simulink model "case8"  (R2024b)
settings: Solver=FixedStepAuto  StartTime=0  StopTime=1  FixedStep=1e-7  RelTol=1e-3
values from neighbouring files (symbols this model uses):
  SG_D_1_D = 0.01056    [IEEE9_case_parameters.m]    (also in case1_parameters.m; case2_parameters.m; case3_parameters.m; case4_parameters.m)
  SG_D_1_EnableSaturation = 0    [IEEE9_case_parameters.m]    (also in case1_parameters.m; case2_parameters.m; case3_parameters.m; case4_parameters.m)
  SG_D_1_f0 = 60    [IEEE9_case_parameters.m]    (also in case1_parameters.m; case2_parameters.m; case3_parameters.m; case4_parameters.m)
  SG_D_1_H = 7.5    [IEEE9_case_parameters.m]    (also in case1_parameters.m; case2_parameters.m; case3_parameters.m; case4_parameters.m)
  SG_D_1_K_A = 20    [IEEE9_case_parameters.m]    (also in case1_parameters.m; case2_parameters.m; case3_parameters.m; case4_parameters.m)
  SG_D_1_K_E = 1.000000e+1    (= 10)    [IEEE9_case_parameters.m]    (also in case1_parameters.m; case2_parameters.m; case3_parameters.m; case4_parameters.m)
  SG_D_1_K_F = 2.363    [IEEE9_case_parameters.m]    (also in case1_parameters.m; case2_parameters.m; case3_parameters.m; case4_parameters.m)
  SG_D_1_K_s = 0.5    [IEEE9_case_parameters.m]    (also in case1_parameters.m = 5; case2_parameters.m = 5; case3_parameters.m = 5; case4_parameters.m = 5)
  SG_D_1_R_a = 0.001088    [IEEE9_case_parameters.m]    (also in case1_parameters.m; case2_parameters.m; case3_parameters.m; case4_parameters.m)
  SG_D_1_S_A = 1    [IEEE9_case_parameters.m]    (also in case1_parameters.m; case2_parameters.m; case3_parameters.m; case4_parameters.m)
  SG_D_1_S_B = 0.103    [IEEE9_case_parameters.m]    (also in case1_parameters.m; case2_parameters.m; case3_parameters.m; case4_parameters.m)
  SG_D_1_S_N = 10.659857    [IEEE9_case_parameters.m]    (also in case1_parameters.m; case2_parameters.m; case3_parameters.m; case4_parameters.m)
  SG_D_1_SpeedPara = 200    [IEEE9_case_parameters.m]    (also in case1_parameters.m; case2_parameters.m; case3_parameters.m; case4_parameters.m)
  SG_D_1_T_0 = 0.720173    [IEEE9_case_parameters.m]    (also in case1_parameters.m = 0.755522; case2_parameters.m = 0.808931; case3_parameters.m = 0.869402; case4_parameters.m = 0.729316)
  SG_D_1_T_1 = 0.3    [IEEE9_case_parameters.m]    (also in case1_parameters.m; case2_parameters.m; case3_parameters.m; case4_parameters.m)
  SG_D_1_T_2 = 0.05    [IEEE9_case_parameters.m]    (also in case1_parameters.m; case2_parameters.m; case3_parameters.m; case4_parameters.m)
  SG_D_1_T_3 = 0.02    [IEEE9_case_parameters.m]    (also in case1_parameters.m; case2_parameters.m; case3_parameters.m; case4_parameters.m)
  SG_D_1_T_4 = 0.005    [IEEE9_case_parameters.m]    (also in case1_parameters.m; case2_parameters.m; case3_parameters.m; case4_parameters.m)
  SG_D_1_T_A = 0.02    [IEEE9_case_parameters.m]    (also in case1_parameters.m; case2_parameters.m; case3_parameters.m; case4_parameters.m)
  SG_D_1_T_dd = 8.000000e+0    (= 8)    [IEEE9_case_parameters.m]    (also in case1_parameters.m; case2_parameters.m; case3_parameters.m; case4_parameters.m)
  SG_D_1_T_ddd = 0.04    [IEEE9_case_parameters.m]    (also in case1_parameters.m; case2_parameters.m; case3_parameters.m; case4_parameters.m)
  SG_D_1_T_E = 0.314    [IEEE9_case_parameters.m]    (also in case1_parameters.m; case2_parameters.m; case3_parameters.m; case4_parameters.m)
  SG_D_1_T_F = 0.35    [IEEE9_case_parameters.m]    (also in case1_parameters.m; case2_parameters.m; case3_parameters.m; case4_parameters.m)
  SG_D_1_T_qd = 0.8    [IEEE9_case_parameters.m]    (also in case1_parameters.m; case2_parameters.m; case3_parameters.m; case4_parameters.m)
  SG_D_1_T_qdd = 0.02    [IEEE9_case_parameters.m]    (also in case1_parameters.m; case2_parameters.m; case3_parameters.m; case4_parameters.m)
  SG_D_1_T_speed = 0.1    [IEEE9_case_parameters.m]    (also in case1_parameters.m = 200; case2_parameters.m = 200; case3_parameters.m = 200; case4_parameters.m = 200)
  SG_D_1_T_w = 0.5    [IEEE9_case_parameters.m]    (also in case1_parameters.m; case2_parameters.m; case3_parameters.m; case4_parameters.m)
  SG_D_1_V_ref = 1.990276    [IEEE9_case_parameters.m]    (also in case1_parameters.m = 2.042296; case2_parameters.m = 2.051388; case3_parameters.m = 2.089584; case4_parameters.m = 2.01845)
  SG_D_1_w_ref = 376.991118    [IEEE9_case_parameters.m]    (also in case1_parameters.m; case2_parameters.m; case3_parameters.m; case4_parameters.m)
  SG_D_1_wb = 6.000000e+1    (= 60)    [IEEE9_case_parameters.m]    (also in case1_parameters.m; case2_parameters.m; case3_parameters.m; case4_parameters.m)
  SG_D_1_x_d = 1.9    [IEEE9_case_parameters.m]    (also in case1_parameters.m; case2_parameters.m; case3_parameters.m; case4_parameters.m)
  SG_D_1_x_dd = 0.302    [IEEE9_case_parameters.m]    (also in case1_parameters.m; case2_parameters.m; case3_parameters.m; case4_parameters.m)
  SG_D_1_x_ddd = 0.204    [IEEE9_case_parameters.m]    (also in case1_parameters.m; case2_parameters.m; case3_parameters.m; case4_parameters.m)
  SG_D_1_x_l = 0.05    [IEEE9_case_parameters.m]    (also in case1_parameters.m; case2_parameters.m; case3_parameters.m; case4_parameters.m)
  SG_D_1_x_q = 1.3    [IEEE9_case_parameters.m]    (also in case1_parameters.m; case2_parameters.m; case3_parameters.m; case4_parameters.m)
  SG_D_1_x_qd = 0.5    [IEEE9_case_parameters.m]    (also in case1_parameters.m; case2_parameters.m; case3_parameters.m; case4_parameters.m)
  SG_D_1_x_qdd = 0.3    [IEEE9_case_parameters.m]    (also in case1_parameters.m; case2_parameters.m; case3_parameters.m; case4_parameters.m)
  SG_D_2_D = 0.02    [IEEE9_case_parameters.m]    (also in case1_parameters.m; case2_parameters.m; case3_parameters.m; case4_parameters.m)
  SG_D_2_EnableSaturation = 0    [IEEE9_case_parameters.m]    (also in case1_parameters.m; case2_parameters.m; case3_parameters.m; case4_parameters.m)
  SG_D_2_f0 = 60    [IEEE9_case_parameters.m]    (also in case1_parameters.m; case2_parameters.m; case3_parameters.m; case4_parameters.m)
  SG_D_2_H = 8.000000e+0    (= 8)    [IEEE9_case_parameters.m]    (also in case1_parameters.m; case2_parameters.m; case3_parameters.m; case4_parameters.m)
  SG_D_2_K_A = 20    [IEEE9_case_parameters.m]    (also in case1_parameters.m; case2_parameters.m; case3_parameters.m; case4_parameters.m)
  SG_D_2_K_E = 1.000000e+1    (= 10)    [IEEE9_case_parameters.m]    (also in case1_parameters.m; case2_parameters.m; case3_parameters.m; case4_parameters.m)
  SG_D_2_K_F = 2.363    [IEEE9_case_parameters.m]    (also in case1_parameters.m; case2_parameters.m; case3_parameters.m; case4_parameters.m)
  SG_D_2_K_s = 0.5    [IEEE9_case_parameters.m]    (also in case1_parameters.m = 4; case2_parameters.m = 4; case3_parameters.m = 4; case4_parameters.m = 4)
  SG_D_2_R_a = 0.001088    [IEEE9_case_parameters.m]    (also in case1_parameters.m; case2_parameters.m; case3_parameters.m; case4_parameters.m)
  SG_D_2_S_A = 1    [IEEE9_case_parameters.m]    (also in case1_parameters.m; case2_parameters.m; case3_parameters.m; case4_parameters.m)
  SG_D_2_S_B = 0.103    [IEEE9_case_parameters.m]    (also in case1_parameters.m; case2_parameters.m; case3_parameters.m; case4_parameters.m)
  SG_D_2_S_N = 10.659857    [IEEE9_case_parameters.m]    (also in case1_parameters.m; case2_parameters.m; case3_parameters.m; case4_parameters.m)
  SG_D_2_SpeedPara = 200    [IEEE9_case_parameters.m]    (also in case1_parameters.m; case2_parameters.m; case3_parameters.m; case4_parameters.m)
  SG_D_2_T_0 = 1.632913    [IEEE9_case_parameters.m]    (also in case1_parameters.m = 1.632925; case2_parameters.m = 1.632915; case3_parameters.m = 1.632914; case4_parameters.m = 1.632927)
  SG_D_2_T_1 = 0.2    [IEEE9_case_parameters.m]    (also in case1_parameters.m; case2_parameters.m; case3_parameters.m; case4_parameters.m)
  SG_D_2_T_2 = 0.05    [IEEE9_case_parameters.m]    (also in case1_parameters.m; case2_parameters.m; case3_parameters.m; case4_parameters.m)
  SG_D_2_T_3 = 0.02    [IEEE9_case_parameters.m]    (also in case1_parameters.m; case2_parameters.m; case3_parameters.m; case4_parameters.m)
  SG_D_2_T_4 = 0.005    [IEEE9_case_parameters.m]    (also in case1_parameters.m; case2_parameters.m; case3_parameters.m; case4_parameters.m)
  SG_D_2_T_A = 0.02    [IEEE9_case_parameters.m]    (also in case1_parameters.m; case2_parameters.m; case3_parameters.m; case4_parameters.m)
  SG_D_2_T_dd = 7.9    [IEEE9_case_parameters.m]    (also in case1_parameters.m; case2_parameters.m; case3_parameters.m; case4_parameters.m)
  SG_D_2_T_ddd = 0.04    [IEEE9_case_parameters.m]    (also in case1_parameters.m; case2_parameters.m; case3_parameters.m; case4_parameters.m)
  SG_D_2_T_E = 0.314    [IEEE9_case_parameters.m]    (also in case1_parameters.m; case2_parameters.m; case3_parameters.m; case4_parameters.m)
  SG_D_2_T_F = 0.35    [IEEE9_case_parameters.m]    (also in case1_parameters.m; case2_parameters.m; case3_parameters.m; case4_parameters.m)
  SG_D_2_T_qd = 0.8    [IEEE9_case_parameters.m]    (also in case1_parameters.m; case2_parameters.m; case3_parameters.m; case4_parameters.m)
  SG_D_2_T_qdd = 0.015    [IEEE9_case_parameters.m]    (also in case1_parameters.m; case2_parameters.m; case3_parameters.m; case4_parameters.m)
  SG_D_2_T_speed = 0.1    [IEEE9_case_parameters.m]    (also in case1_parameters.m = 150; case2_parameters.m = 150; case3_parameters.m = 150; case4_parameters.m = 150)
  SG_D_2_T_w = 0.35    [IEEE9_case_parameters.m]    (also in case1_parameters.m; case2_parameters.m; case3_parameters.m; case4_parameters.m)
  SG_D_2_V_ref = 2.58547    [IEEE9_case_parameters.m]    (also in case1_parameters.m = 2.597896; case2_parameters.m = 2.587136; case3_parameters.m = 2.586042; case4_parameters.m = 2.599679)
  SG_D_2_w_ref = 376.991118    [IEEE9_case_parameters.m]    (also in case1_parameters.m; case2_parameters.m; case3_parameters.m; case4_parameters.m)
  SG_D_2_wb = 6.000000e+1    (= 60)    [IEEE9_case_parameters.m]    (also in case1_parameters.m; case2_parameters.m; case3_parameters.m; case4_parameters.m)
  SG_D_2_x_d = 1.8    [IEEE9_case_parameters.m]    (also in case1_parameters.m; case2_parameters.m; case3_parameters.m; case4_parameters.m)
  SG_D_2_x_dd = 0.302    [IEEE9_case_parameters.m]    (also in case1_parameters.m; case2_parameters.m; case3_parameters.m; case4_parameters.m)
  SG_D_2_x_ddd = 0.204    [IEEE9_case_parameters.m]    (also in case1_parameters.m; case2_parameters.m; case3_parameters.m; case4_parameters.m)
  SG_D_2_x_l = 0.05    [IEEE9_case_parameters.m]    (also in case1_parameters.m; case2_parameters.m; case3_parameters.m; case4_parameters.m)
  SG_D_2_x_q = 1.25    [IEEE9_case_parameters.m]    (also in case1_parameters.m; case2_parameters.m; case3_parameters.m; case4_parameters.m)
  SG_D_2_x_qd = 0.5    [IEEE9_case_parameters.m]    (also in case1_parameters.m; case2_parameters.m; case3_parameters.m; case4_parameters.m)
  SG_D_2_x_qdd = 0.3    [IEEE9_case_parameters.m]    (also in case1_parameters.m; case2_parameters.m; case3_parameters.m; case4_parameters.m)
  SG_D_3_D = 0.02    [IEEE9_case_parameters.m]    (also in case1_parameters.m; case2_parameters.m; case3_parameters.m; case4_parameters.m)
  SG_D_3_EnableSaturation = 0    [IEEE9_case_parameters.m]    (also in case1_parameters.m; case2_parameters.m; case3_parameters.m; case4_parameters.m)
  SG_D_3_f0 = 60    [IEEE9_case_parameters.m]    (also in case1_parameters.m; case2_parameters.m; case3_parameters.m; case4_parameters.m)
  SG_D_3_H = 7.7    [IEEE9_case_parameters.m]    (also in case1_parameters.m; case2_parameters.m; case3_parameters.m; case4_parameters.m)
  SG_D_3_K_A = 20    [IEEE9_case_parameters.m]    (also in case1_parameters.m; case2_parameters.m; case3_parameters.m; case4_parameters.m)
  SG_D_3_K_E = 1.000000e+1    (= 10)    [IEEE9_case_parameters.m]    (also in case1_parameters.m; case2_parameters.m; case3_parameters.m; case4_parameters.m)
  SG_D_3_K_F = 2.363    [IEEE9_case_parameters.m]    (also in case1_parameters.m; case2_parameters.m; case3_parameters.m; case4_parameters.m)
  SG_D_3_K_s = 0.2    [IEEE9_case_parameters.m]    (also in case1_parameters.m = 2; case2_parameters.m = 2; case3_parameters.m = 2; case4_parameters.m = 2)
  SG_D_3_R_a = 0.001088    [IEEE9_case_parameters.m]    (also in case1_parameters.m; case2_parameters.m; case3_parameters.m; case4_parameters.m)
  SG_D_3_S_A = 1    [IEEE9_case_parameters.m]    (also in case1_parameters.m; case2_parameters.m; case3_parameters.m; case4_parameters.m)
  SG_D_3_S_B = 0.103    [IEEE9_case_parameters.m]    (also in case1_parameters.m; case2_parameters.m; case3_parameters.m; case4_parameters.m)
  SG_D_3_S_N = 10.659857    [IEEE9_case_parameters.m]    (also in case1_parameters.m; case2_parameters.m; case3_parameters.m; case4_parameters.m)
  SG_D_3_SpeedPara = 200    [IEEE9_case_parameters.m]    (also in case1_parameters.m; case2_parameters.m; case3_parameters.m; case4_parameters.m)
  SG_D_3_T_0 = 0.850788    [IEEE9_case_parameters.m]    (also in case1_parameters.m = 0.850786; case2_parameters.m = 0.850787; case3_parameters.m; case4_parameters.m = 0.850786)
  SG_D_3_T_1 = 0.2    [IEEE9_case_parameters.m]    (also in case1_parameters.m; case2_parameters.m; case3_parameters.m; case4_parameters.m)
  SG_D_3_T_2 = 0.05    [IEEE9_case_parameters.m]    (also in case1_parameters.m; case2_parameters.m; case3_parameters.m; case4_parameters.m)
  SG_D_3_T_3 = 0.02    [IEEE9_case_parameters.m]    (also in case1_parameters.m; case2_parameters.m; case3_parameters.m; case4_parameters.m)
  SG_D_3_T_4 = 0.005    [IEEE9_case_parameters.m]    (also in case1_parameters.m; case2_parameters.m; case3_parameters.m; case4_parameters.m)
  SG_D_3_T_A = 0.02    [IEEE9_case_parameters.m]    (also in case1_parameters.m; case2_parameters.m; case3_parameters.m; case4_parameters.m)
  SG_D_3_T_dd = 8.1    [IEEE9_case_parameters.m]    (also in case1_parameters.m; case2_parameters.m; case3_parameters.m; case4_parameters.m)
  SG_D_3_T_ddd = 0.04    [IEEE9_case_parameters.m]    (also in case1_parameters.m; case2_parameters.m; case3_parameters.m; case4_parameters.m)
  SG_D_3_T_E = 0.314    [IEEE9_case_parameters.m]    (also in case1_parameters.m; case2_parameters.m; case3_parameters.m; case4_parameters.m)
  SG_D_3_T_F = 0.35    [IEEE9_case_parameters.m]    (also in case1_parameters.m; case2_parameters.m; case3_parameters.m; case4_parameters.m)
  SG_D_3_T_qd = 0.8    [IEEE9_case_parameters.m]    (also in case1_parameters.m; case2_parameters.m; case3_parameters.m; case4_parameters.m)
  SG_D_3_T_qdd = 0.015    [IEEE9_case_parameters.m]    (also in case1_parameters.m; case2_parameters.m; case3_parameters.m; case4_parameters.m)
  SG_D_3_T_speed = 0.1    [IEEE9_case_parameters.m]    (also in case1_parameters.m = 180; case2_parameters.m = 180; case3_parameters.m = 180; case4_parameters.m = 180)
  SG_D_3_T_w = 0.4    [IEEE9_case_parameters.m]    (also in case1_parameters.m; case2_parameters.m; case3_parameters.m; case4_parameters.m)
  SG_D_3_V_ref = 1.892727    [IEEE9_case_parameters.m]    (also in case1_parameters.m = 1.906439; case2_parameters.m = 1.895535; case3_parameters.m = 1.892105; case4_parameters.m = 1.906598)
  SG_D_3_w_ref = 376.991118    [IEEE9_case_parameters.m]    (also in case1_parameters.m; case2_parameters.m; case3_parameters.m; case4_parameters.m)
  SG_D_3_wb = 6.000000e+1    (= 60)    [IEEE9_case_parameters.m]    (also in case1_parameters.m; case2_parameters.m; case3_parameters.m; case4_parameters.m)
  SG_D_3_x_d = 1.85    [IEEE9_case_parameters.m]    (also in case1_parameters.m; case2_parameters.m; case3_parameters.m; case4_parameters.m)
  SG_D_3_x_dd = 0.302    [IEEE9_case_parameters.m]    (also in case1_parameters.m; case2_parameters.m; case3_parameters.m; case4_parameters.m)
  SG_D_3_x_ddd = 0.204    [IEEE9_case_parameters.m]    (also in case1_parameters.m; case2_parameters.m; case3_parameters.m; case4_parameters.m)
  SG_D_3_x_l = 0.05    [IEEE9_case_parameters.m]    (also in case1_parameters.m; case2_parameters.m; case3_parameters.m; case4_parameters.m)
  SG_D_3_x_q = 1.2    [IEEE9_case_parameters.m]    (also in case1_parameters.m; case2_parameters.m; case3_parameters.m; case4_parameters.m)
  SG_D_3_x_qd = 0.5    [IEEE9_case_parameters.m]    (also in case1_parameters.m; case2_parameters.m; case3_parameters.m; case4_parameters.m)
  SG_D_3_x_qdd = 0.3    [IEEE9_case_parameters.m]    (also in case1_parameters.m; case2_parameters.m; case3_parameters.m; case4_parameters.m)
(part 11 of 12)

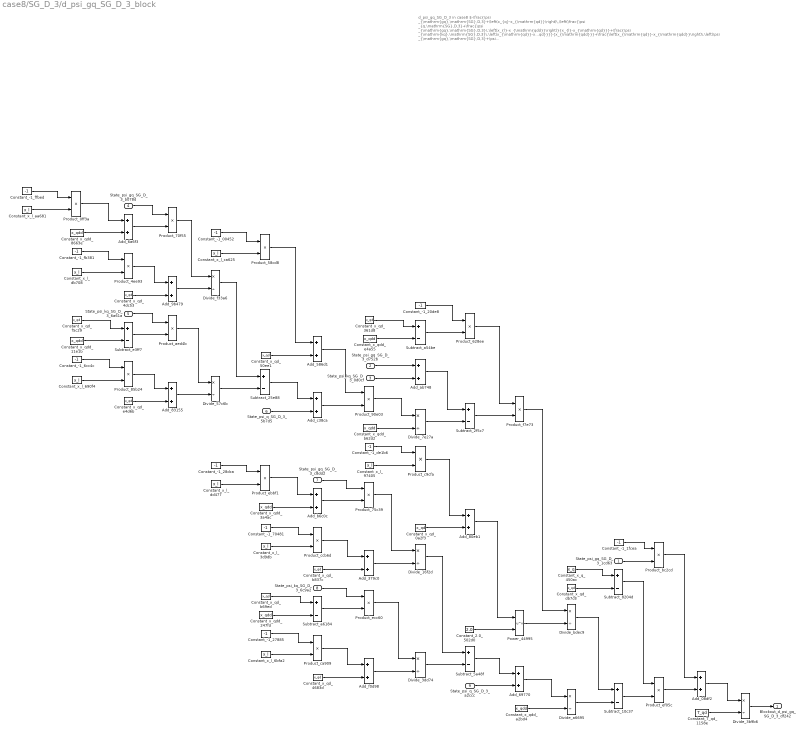
== system case8/SG_D_3/d_psi_gq_SG_D_3_block ==
  note: d_psi_gq_SG_D_3 in case8
      | $-\frac{\psi _{\mathrm{gq},\mathrm{SG},D,3}+\left(x_{q}-x_{\mathrm{qd}}\right)\,\left(\frac{\psi _{q,\mathrm{SG},D,3}+\frac{\psi _{\mathrm{gq},\mathrm{SG},D,3}\,\left(x_{l}-x_{\mathrm{qdd}}\right)}{x_{l}-x_{\mathrm{qd}}}+\frac{\psi _{\mathrm{kq},\mathrm{SG},D,3}\,\left(x_{\mathrm{qd}}-x_{\mathrm{qdd}}\right)}{x_{l}-x_{\mathrm{qd}}}}{x_{\mathrm{qdd}}}+\frac{\left(x_{\mathrm{qd}}-x_{\mathrm{qdd}}\right)\,\left(\psi _{\mathrm{gq},\mathrm{SG},D,3}+\psi _{\mathrm{kq},\mathrm{SG},D,3}+\frac{\left(x_{l}-x_{\mathrm{qd}}\right)\,\left(\psi _{q,\mathrm{SG},D,3}+\frac{\psi _{\mathrm{gq},\mathrm{SG},D,3}\,\left(x_{l}-x_{\mathrm{qdd}}\right)}{x_{l}-x_{\mathrm{qd}}}+\frac{\psi _{\mathrm{kq},\mathrm{SG},D,3}\,\left(x_{\mathrm{qd}}-x_{\mathrm{qdd}}\right)}{x_{l}-x_{\mathrm{qd}}}\right)}{x_{\mathrm{qdd}}}\right)}{{\left(x_{l}-x_{\mathrm{qd}}\right)}^2}\right)}{T_{\mathrm{qd}}}$
      | Automatically generated on 2025-10-31 19:30:10 .
  State_psi_gq_SG_D_3_1cd63 : Inport
  State_psi_gq_SG_D_3_d752b : Inport  Port=2
  State_psi_kq_SG_D_3_0d0cf : Inport  Port=3
  State_psi_gq_SG_D_3_b078d : Inport  Port=4
  State_psi_kq_SG_D_3_6a61a : Inport  Port=5
  State_psi_q_SG_D_3_5b7d5 : Inport  Port=6
  State_psi_gq_SG_D_3_c8dd2 : Inport  Port=7
  State_psi_kq_SG_D_3_6c9a2 : Inport  Port=8
  State_psi_q_SG_D_3_a2ccc : Inport  Port=9
  Add_08df2 : Sum
  Add_379c0 : Sum
  Add_586d1 : Sum
  Add_69770 : Sum
  Add_6a6f3 : Sum
  Add_80eb1 : Sum
  Add_83155 : Sum
  Add_9b479 : Sum
  Add_ab748 : Sum
  Add_b6c0c : Sum
  Add_c38ca : Sum
  Add_f0d98 : Sum
  Constant_-1_00452 : Constant  Value=-1
  Constant_-1_1fcea : Constant  Value=-1
  Constant_-1_20de8 : Constant  Value=-1
  Constant_-1_27885 : Constant  Value=-1
  Constant_-1_28dca : Constant  Value=-1
  Constant_-1_6cc4c : Constant  Value=-1
  Constant_-1_70481 : Constant  Value=-1
  Constant_-1_de1b6 : Constant  Value=-1
  Constant_-1_fb381 : Constant  Value=-1
  Constant_-1_ffbed : Constant  Value=-1
  Constant_2.0_502d0 : Constant  Value=2.0
  Constant_T_qd_1158e : Constant  Value=T_qd
  Constant_x_l_3d9db : Constant  Value=x_l
  Constant_x_l_690f4 : Constant  Value=x_l
  Constant_x_l_6bfa2 : Constant  Value=x_l
  Constant_x_l_97405 : Constant  Value=x_l
  Constant_x_l_aa681 : Constant  Value=x_l
  Constant_x_l_ca625 : Constant  Value=x_l
  Constant_x_l_db708 : Constant  Value=x_l
  Constant_x_l_dd477 : Constant  Value=x_l
  Constant_x_q_450ac : Constant  Value=x_q
  Constant_x_qd_0a2f3 : Constant  Value=x_qd
  Constant_x_qd_361d8 : Constant  Value=x_qd
  Constant_x_qd_4683d : Constant  Value=x_qd
  Constant_x_qd_4dc53 : Constant  Value=x_qd
  Constant_x_qd_50ee1 : Constant  Value=x_qd
  Constant_x_qd_b69ed : Constant  Value=x_qd
  Constant_x_qd_b837c : Constant  Value=x_qd
  Constant_x_qd_db7c8 : Constant  Value=x_qd
  Constant_x_qd_e4d6b : Constant  Value=x_qd
  Constant_x_qd_f5c29 : Constant  Value=x_qd
  Constant_x_qdd_11e1b : Constant  Value=x_qdd
  Constant_x_qdd_247fd : Constant  Value=x_qdd
  Constant_x_qdd_3a4ac : Constant  Value=x_qdd
  Constant_x_qdd_8663e : Constant  Value=x_qdd
  Constant_x_qdd_a2bd4 : Constant  Value=x_qdd
  Constant_x_qdd_b62d2 : Constant  Value=x_qdd
  Constant_x_qdd_e4a55 : Constant  Value=x_qdd
  Divide_16f2d : Product  Inputs=*/
  Divide_3b9b6 : Product  Inputs=*/
  Divide_3dd74 : Product  Inputs=*/
  Divide_57c6b : Product  Inputs=*/
  Divide_7e27a : Product  Inputs=*/
  Divide_a6695 : Product  Inputs=*/
  Divide_bdec9 : Product  Inputs=*/
  Divide_f33a6 : Product  Inputs=*/
  Power_44995 : Math  Operator=pow
  Product_0ff3a : Product
  Product_4ee93 : Product
  Product_58cd8 : Product
  Product_628ee : Product
  Product_70f55 : Product
  Product_75c39 : Product
  Product_85b24 : Product
  Product_90e03 : Product
  Product_aed4b : Product
  Product_bc2cd : Product
  Product_c9cfa : Product
  Product_ca909 : Product
  Product_ccb6d : Product
  Product_ebbf1 : Product
  Product_ecc60 : Product
  Product_ef05c : Product
  Product_f7e73 : Product
  Subtract_10c37 : Sum  Inputs=+-
  Subtract_25e88 : Sum  Inputs=+-
  Subtract_2f5c7 : Sum  Inputs=+-
  Subtract_5a48f : Sum  Inputs=+-
  Subtract_8204d : Sum  Inputs=+-
  Subtract_a54be : Sum  Inputs=+-
  Subtract_a6184 : Sum  Inputs=+-
  Subtract_e3ff7 : Sum  Inputs=+-
  Blockout_d_psi_gq_SG_D_3_df242 : Outport
  wires:
  Constant_x_l_97405/1 -> Product_c9cfa/2
  Constant_x_qd_f5c29/1 -> Subtract_e3ff7/1
  Add_586d1/1 -> Product_90e03/1
  Constant_-1_ffbed/1 -> Product_0ff3a/1
  Add_6a6f3/1 -> Product_70f55/2
  Constant_x_qdd_11e1b/1 -> Subtract_e3ff7/2
  Constant_x_qd_50ee1/1 -> Add_586d1/2
  Constant_x_l_aa681/1 -> Product_0ff3a/2
  Constant_x_l_db708/1 -> Product_4ee93/2
  Add_f0d98/1 -> Divide_3dd74/2
  State_psi_kq_SG_D_3_0d0cf/1 -> Add_ab748/2
  Constant_x_qdd_8663e/1 -> Add_6a6f3/2
  Product_0ff3a/1 -> Add_6a6f3/1
  Constant_x_qd_4683d/1 -> Add_f0d98/2
  Product_628ee/1 -> Product_f7e73/1
  Constant_-1_28dca/1 -> Product_ebbf1/1
  Constant_-1_fb381/1 -> Product_4ee93/1
  Constant_-1_6cc4c/1 -> Product_85b24/1
  Constant_x_l_690f4/1 -> Product_85b24/2
  Constant_-1_20de8/1 -> Product_628ee/1
  Constant_-1_1fcea/1 -> Product_bc2cd/1
  State_psi_gq_SG_D_3_b078d/1 -> Product_70f55/1
  Product_ebbf1/1 -> Add_b6c0c/1
  Product_4ee93/1 -> Add_9b479/1
  Product_ca909/1 -> Add_f0d98/1
  Constant_x_qd_4dc53/1 -> Add_9b479/2
  Constant_-1_70481/1 -> Product_ccb6d/1
  State_psi_kq_SG_D_3_6a61a/1 -> Product_aed4b/1
  Subtract_e3ff7/1 -> Product_aed4b/2
  Product_85b24/1 -> Add_83155/1
  Add_b6c0c/1 -> Product_75c39/2
  Add_9b479/1 -> Divide_f33a6/2
  Constant_x_qd_e4d6b/1 -> Add_83155/2
  Product_70f55/1 -> Divide_f33a6/1
  Constant_T_qd_1158e/1 -> Divide_3b9b6/2
  Product_ccb6d/1 -> Add_379c0/1
  Product_aed4b/1 -> Divide_57c6b/1
  Product_ecc60/1 -> Divide_3dd74/1
  Add_83155/1 -> Divide_57c6b/2
  Constant_-1_00452/1 -> Product_58cd8/1
  Constant_x_qdd_b62d2/1 -> Divide_7e27a/2
  Constant_x_l_ca625/1 -> Product_58cd8/2
  Divide_f33a6/1 -> Subtract_25e88/1
  Constant_x_qd_db7c8/1 -> Subtract_8204d/2
  Add_379c0/1 -> Divide_16f2d/2
  Divide_57c6b/1 -> Subtract_25e88/2
  Constant_x_l_dd477/1 -> Product_ebbf1/2
  Product_58cd8/1 -> Add_586d1/1
  Constant_-1_de1b6/1 -> Product_c9cfa/1
  Constant_x_l_3d9db/1 -> Product_ccb6d/2
  Subtract_25e88/1 -> Add_c38ca/1
  State_psi_q_SG_D_3_5b7d5/1 -> Add_c38ca/2
  Constant_-1_27885/1 -> Product_ca909/1
  Constant_x_qdd_3a4ac/1 -> Add_b6c0c/2
  Constant_x_qd_b69ed/1 -> Subtract_a6184/1
  Constant_x_qdd_247fd/1 -> Subtract_a6184/2
  Constant_x_l_6bfa2/1 -> Product_ca909/2
  Add_c38ca/1 -> Product_90e03/2
  Constant_x_qdd_e4a55/1 -> Subtract_a54be/2
  State_psi_gq_SG_D_3_c8dd2/1 -> Product_75c39/1
  Constant_x_qd_b837c/1 -> Add_379c0/2
  Divide_bdec9/1 -> Subtract_10c37/1
  State_psi_kq_SG_D_3_6c9a2/1 -> Product_ecc60/1
  Subtract_a6184/1 -> Product_ecc60/2
  Constant_x_qd_361d8/1 -> Subtract_a54be/1
  State_psi_gq_SG_D_3_d752b/1 -> Add_ab748/1
  Product_90e03/1 -> Divide_7e27a/1
  Product_75c39/1 -> Divide_16f2d/1
  Subtract_a54be/1 -> Product_628ee/2
  Add_ab748/1 -> Subtract_2f5c7/1
  Divide_7e27a/1 -> Subtract_2f5c7/2
  Product_c9cfa/1 -> Add_80eb1/1
  Constant_x_qd_0a2f3/1 -> Add_80eb1/2
  Divide_16f2d/1 -> Subtract_5a48f/1
  Divide_3dd74/1 -> Subtract_5a48f/2
  Subtract_2f5c7/1 -> Product_f7e73/2
  Add_80eb1/1 -> Power_44995/1
  Constant_2.0_502d0/1 -> Power_44995/2
  Subtract_5a48f/1 -> Add_69770/1
  State_psi_q_SG_D_3_a2ccc/1 -> Add_69770/2
  Product_f7e73/1 -> Divide_bdec9/1
  Power_44995/1 -> Divide_bdec9/2
  Add_69770/1 -> Divide_a6695/1
  Constant_x_qdd_a2bd4/1 -> Divide_a6695/2
  Constant_x_q_450ac/1 -> Subtract_8204d/1
  Divide_a6695/1 -> Subtract_10c37/2
  State_psi_gq_SG_D_3_1cd63/1 -> Product_bc2cd/2
  Subtract_8204d/1 -> Product_ef05c/1
  Subtract_10c37/1 -> Product_ef05c/2
  Product_bc2cd/1 -> Add_08df2/1
  Product_ef05c/1 -> Add_08df2/2
  Add_08df2/1 -> Divide_3b9b6/1
  Divide_3b9b6/1 -> Blockout_d_psi_gq_SG_D_3_df242/1

== system case8/SG_D_3/d_psi_kq_SG_D_3_block ==
  note: d_psi_kq_SG_D_3 in case8
      | $-\frac{\psi _{\mathrm{gq},\mathrm{SG},D,3}+\psi _{\mathrm{kq},\mathrm{SG},D,3}+\frac{\left(x_{l}-x_{\mathrm{qd}}\right)\,\left(\psi _{q,\mathrm{SG},D,3}+\frac{\psi _{\mathrm{gq},\mathrm{SG},D,3}\,\left(x_{l}-x_{\mathrm{qdd}}\right)}{x_{l}-x_{\mathrm{qd}}}+\frac{\psi _{\mathrm{kq},\mathrm{SG},D,3}\,\left(x_{\mathrm{qd}}-x_{\mathrm{qdd}}\right)}{x_{l}-x_{\mathrm{qd}}}\right)}{x_{\mathrm{qdd}}}}{T_{\mathrm{qdd}}}$
      | Automatically generated on 2025-10-31 19:30:11 .
  State_psi_gq_SG_D_3_1d67a : Inport
  State_psi_kq_SG_D_3_44aa7 : Inport  Port=2
  State_psi_gq_SG_D_3_6d3fb : Inport  Port=3
  State_psi_kq_SG_D_3_0268c : Inport  Port=4
  State_psi_q_SG_D_3_9bd31 : Inport  Port=5
  Add_0695f : Sum
  Add_8a3c0 : Sum
  Add_a7f02 : Sum
  Add_ad730 : Sum
  Add_d3057 : Sum
  Add_e76be : Sum
  Constant_-1_56ca5 : Constant  Value=-1
  Constant_-1_756ca : Constant  Value=-1
  Constant_-1_77a47 : Constant  Value=-1
  Constant_-1_960c4 : Constant  Value=-1
  Constant_-1_e4aac : Constant  Value=-1
  Constant_T_qdd_24111 : Constant  Value=T_qdd
  Constant_x_l_4c7c5 : Constant  Value=x_l
  Constant_x_l_eade0 : Constant  Value=x_l
  Constant_x_l_efded : Constant  Value=x_l
  Constant_x_l_fbfc4 : Constant  Value=x_l
  Constant_x_qd_39cd4 : Constant  Value=x_qd
  Constant_x_qd_7849f : Constant  Value=x_qd
  Constant_x_qd_a575e : Constant  Value=x_qd
  Constant_x_qd_c6d55 : Constant  Value=x_qd
  Constant_x_qdd_8cdb3 : Constant  Value=x_qdd
  Constant_x_qdd_ad474 : Constant  Value=x_qdd
  Constant_x_qdd_f0d6c : Constant  Value=x_qdd
  Divide_010a2 : Product  Inputs=*/
  Divide_357f7 : Product  Inputs=*/
  Divide_7ee2a : Product  Inputs=*/
  Divide_d0a17 : Product  Inputs=*/
  Product_091dc : Product
  Product_0ecf1 : Product
  Product_146d4 : Product
  Product_19748 : Product
  Product_5a058 : Product
  Product_60277 : Product
  Product_b83d4 : Product
  Product_ec5aa : Product
  Subtract_1fdec : Sum  Inputs=+-
  Subtract_45c9f : Sum  Inputs=+-
  Subtract_6abec : Sum  Inputs=+-
  Blockout_d_psi_kq_SG_D_3_6329c : Outport
  wires:
  State_psi_q_SG_D_3_9bd31/1 -> Add_0695f/2
  Constant_-1_56ca5/1 -> Product_5a058/1
  Constant_-1_77a47/1 -> Product_b83d4/1
  Constant_-1_756ca/1 -> Product_0ecf1/1
  Constant_x_l_fbfc4/1 -> Product_5a058/2
  Constant_x_qdd_f0d6c/1 -> Add_d3057/2
  Product_19748/1 -> Add_a7f02/1
  Constant_x_l_efded/1 -> Product_b83d4/2
  Constant_x_qd_39cd4/1 -> Subtract_6abec/1
  Product_b83d4/1 -> Add_d3057/1
  Constant_x_l_eade0/1 -> Product_091dc/2
  Constant_x_qdd_8cdb3/1 -> Subtract_6abec/2
  Constant_-1_e4aac/1 -> Product_19748/1
  Constant_x_l_4c7c5/1 -> Product_19748/2
  State_psi_gq_SG_D_3_6d3fb/1 -> Product_ec5aa/1
  Add_d3057/1 -> Product_ec5aa/2
  Add_0695f/1 -> Product_60277/2
  Product_5a058/1 -> Add_ad730/1
  Constant_x_qd_c6d55/1 -> Add_ad730/2
  State_psi_kq_SG_D_3_0268c/1 -> Product_146d4/1
  Subtract_6abec/1 -> Product_146d4/2
  Add_ad730/1 -> Divide_010a2/2
  Constant_x_qd_a575e/1 -> Add_a7f02/2
  Product_ec5aa/1 -> Divide_010a2/1
  Product_146d4/1 -> Divide_d0a17/1
  Add_a7f02/1 -> Divide_d0a17/2
  Constant_-1_960c4/1 -> Product_091dc/1
  Divide_010a2/1 -> Subtract_45c9f/1
  Add_8a3c0/1 -> Divide_7ee2a/1
  Divide_d0a17/1 -> Subtract_45c9f/2
  Divide_7ee2a/1 -> Blockout_d_psi_kq_SG_D_3_6329c/1
  Product_091dc/1 -> Add_e76be/1
  Constant_x_qd_7849f/1 -> Add_e76be/2
  Subtract_45c9f/1 -> Add_0695f/1
  State_psi_gq_SG_D_3_1d67a/1 -> Product_0ecf1/2
  Add_e76be/1 -> Product_60277/1
  Constant_T_qdd_24111/1 -> Divide_7ee2a/2
  Product_0ecf1/1 -> Subtract_1fdec/1
  State_psi_kq_SG_D_3_44aa7/1 -> Subtract_1fdec/2
  Product_60277/1 -> Divide_357f7/1
  Constant_x_qdd_ad474/1 -> Divide_357f7/2
  Subtract_1fdec/1 -> Add_8a3c0/1
  Divide_357f7/1 -> Add_8a3c0/2

== system case8/SG_D_3/d_psi_q_SG_D_3_block ==
  note: d_psi_q_SG_D_3 in case8
      | $2\,\pi \,f_{0}\,\left(v_{d,\mathrm{SG},D,3}\,\cos\left(\theta _{\mathrm{SG},D,3}\right)+v_{q,\mathrm{SG},D,3}\,\sin\left(\theta _{\mathrm{SG},D,3}\right)-\frac{R_{a}\,\left(\psi _{q,\mathrm{SG},D,3}+\frac{\psi _{\mathrm{gq},\mathrm{SG},D,3}\,\left(x_{l}-x_{\mathrm{qdd}}\right)}{x_{l}-x_{\mathrm{qd}}}+\frac{\psi _{\mathrm{kq},\mathrm{SG},D,3}\,\left(x_{\mathrm{qd}}-x_{\mathrm{qdd}}\right)}{x_{l}-x_{\mathrm{qd}}}\right)}{x_{\mathrm{qdd}}}-\frac{\psi _{d,\mathrm{SG},D,3}\,w_{\mathrm{SG},D,3}}{2\,f_{0}\,\pi }\right)$
      | Automatically generated on 2025-10-31 19:30:06 .
  State_psi_gq_SG_D_3_bc5a9 : Inport
  State_psi_kq_SG_D_3_afd1f : Inport  Port=2
  State_psi_q_SG_D_3_c2b51 : Inport  Port=3
  Input_v_d_SG_D_3_a1afd : Inport  Port=4
  State_theta_SG_D_3_3c006 : Inport  Port=5
  Input_v_q_SG_D_3_3c190 : Inport  Port=6
  State_theta_SG_D_3_65b3a : Inport  Port=7
  State_psi_d_SG_D_3_3d93d : Inport  Port=8
  State_w_SG_D_3_cea80 : Inport  Port=9
  Add_1891b : Sum
  Add_2586e : Sum
  Add_4c63a : Sum
  Add_4fa47 : Sum
  Add_61df1 : Sum
  Constant_-1_24081 : Constant  Value=-1
  Constant_-1_9f161 : Constant  Value=-1
  Constant_-1_d5ee5 : Constant  Value=-1
  Constant_-2.0_fb8a8 : Constant  Value=-2.0
  Constant_2.0_b52c9 : Constant  Value=2.0
  Constant_R_a_d3e9e : Constant  Value=R_a
  Constant_f0_2bf4b : Constant  Value=f0
  Constant_f0_5cd14 : Constant  Value=f0
  Constant_pi_379ce : Constant  Value=pi
  Constant_pi_df045 : Constant  Value=pi
  Constant_x_l_5992e : Constant  Value=x_l
  Constant_x_l_66390 : Constant  Value=x_l
  Constant_x_l_cbf2c : Constant  Value=x_l
  Constant_x_qd_29300 : Constant  Value=x_qd
  Constant_x_qd_b0f1d : Constant  Value=x_qd
  Constant_x_qd_c4ef9 : Constant  Value=x_qd
  Constant_x_qdd_55636 : Constant  Value=x_qdd
  Constant_x_qdd_5eca8 : Constant  Value=x_qdd
  Constant_x_qdd_f9d8f : Constant  Value=x_qdd
  Divide_18857 : Product  Inputs=*/
  Divide_19f1b : Product  Inputs=*/
  Divide_9b1c5 : Product  Inputs=*/
  Divide_d1fa5 : Product  Inputs=*/
  MathFunc_cos_3c322 : Trigonometry  Operator=cos
  MathFunc_sin_1bd6a : Trigonometry
  Product_03b9a : Product
  Product_06b74 : Product
  Product_343a4 : Product
  Product_53b20 : Product
  Product_5dba2 : Product
  Product_5eea5 : Product
  Product_679d7 : Product
  Product_6cc5a : Product
  Product_835df : Product
  Product_8458f : Product
  Product_99844 : Product
  Product_c4e25 : Product
  Product_d3e95 : Product
  Product_ed672 : Product
  Subtract_b0341 : Sum  Inputs=+-
  Subtract_e51e5 : Sum  Inputs=+-
  Subtract_eb0e5 : Sum  Inputs=+-
  Subtract_fade6 : Sum  Inputs=+-
  Blockout_d_psi_q_SG_D_3_2b12b : Outport
  wires:
  Constant_x_qd_b0f1d/1 -> Subtract_eb0e5/1
  Constant_pi_df045/1 -> Product_d3e95/2
  Product_835df/1 -> Divide_18857/1
  Constant_x_l_66390/1 -> Product_343a4/2
  Constant_f0_5cd14/1 -> Product_03b9a/2
  State_w_SG_D_3_cea80/1 -> Product_679d7/2
  Constant_-1_d5ee5/1 -> Product_53b20/1
  Constant_x_qdd_55636/1 -> Add_4fa47/2
  Input_v_d_SG_D_3_a1afd/1 -> Product_99844/1
  Constant_x_qdd_5eca8/1 -> Subtract_eb0e5/2
  Constant_x_l_5992e/1 -> Product_53b20/2
  Divide_9b1c5/1 -> Add_1891b/2
  Product_53b20/1 -> Add_4fa47/1
  Constant_2.0_b52c9/1 -> Product_d3e95/1
  Add_61df1/1 -> Product_835df/2
  Constant_-1_24081/1 -> Product_343a4/1
  Constant_x_qd_29300/1 -> Add_4c63a/2
  Constant_-1_9f161/1 -> Product_5dba2/1
  Subtract_fade6/1 -> Subtract_e51e5/1
  Constant_x_l_cbf2c/1 -> Product_5dba2/2
  Subtract_e51e5/1 -> Add_1891b/1
  Constant_f0_2bf4b/1 -> Product_06b74/2
  State_theta_SG_D_3_65b3a/1 -> MathFunc_sin_1bd6a/1
  Constant_x_qd_c4ef9/1 -> Add_2586e/2
  State_psi_gq_SG_D_3_bc5a9/1 -> Product_6cc5a/1
  Add_4fa47/1 -> Product_6cc5a/2
  Product_d3e95/1 -> Product_06b74/1
  Product_343a4/1 -> Add_2586e/1
  State_psi_kq_SG_D_3_afd1f/1 -> Product_5eea5/1
  Subtract_eb0e5/1 -> Product_5eea5/2
  Product_5dba2/1 -> Add_4c63a/1
  MathFunc_sin_1bd6a/1 -> Product_ed672/2
  Product_6cc5a/1 -> Divide_d1fa5/1
  Product_06b74/1 -> Divide_9b1c5/2
  Add_2586e/1 -> Divide_d1fa5/2
  Product_5eea5/1 -> Divide_19f1b/1
  Add_4c63a/1 -> Divide_19f1b/2
  Input_v_q_SG_D_3_3c190/1 -> Product_ed672/1
  Divide_d1fa5/1 -> Subtract_b0341/1
  Subtract_b0341/1 -> Add_61df1/1
  Divide_19f1b/1 -> Subtract_b0341/2
  Divide_18857/1 -> Subtract_fade6/1
  State_psi_q_SG_D_3_c2b51/1 -> Add_61df1/2
  Product_ed672/1 -> Subtract_e51e5/2
  Constant_R_a_d3e9e/1 -> Product_835df/1
  State_theta_SG_D_3_3c006/1 -> MathFunc_cos_3c322/1
  Constant_x_qdd_f9d8f/1 -> Divide_18857/2
  MathFunc_cos_3c322/1 -> Product_99844/2
  Constant_-2.0_fb8a8/1 -> Product_c4e25/1
  Product_99844/1 -> Subtract_fade6/2
  State_psi_d_SG_D_3_3d93d/1 -> Product_679d7/1
  Constant_pi_379ce/1 -> Product_c4e25/2
  Product_679d7/1 -> Divide_9b1c5/1
  Product_c4e25/1 -> Product_03b9a/1
  Product_03b9a/1 -> Product_8458f/1
  Add_1891b/1 -> Product_8458f/2
  Product_8458f/1 -> Blockout_d_psi_q_SG_D_3_2b12b/1

== system case8/SG_D_3/d_theta_SG_D_3_block ==
  note: d_theta_SG_D_3 in case8
      | $w_{\mathrm{SG},D,3}-2\,\pi \,f_{0}$
      | Automatically generated on 2025-10-31 19:30:12 .
  State_w_SG_D_3_084e9 : Inport
  Add_b36e5 : Sum
  Constant_-2.0_70651 : Constant  Value=-2.0
  Constant_f0_94721 : Constant  Value=f0
  Constant_pi_5638e : Constant  Value=pi
  Product_2d093 : Product
  Product_d28b3 : Product
  Blockout_d_theta_SG_D_3_e0920 : Outport
  wires:
  Constant_-2.0_70651/1 -> Product_d28b3/1
  Constant_pi_5638e/1 -> Product_d28b3/2
  State_w_SG_D_3_084e9/1 -> Add_b36e5/2
  Product_d28b3/1 -> Product_2d093/1
  Constant_f0_94721/1 -> Product_2d093/2
  Product_2d093/1 -> Add_b36e5/1
  Add_b36e5/1 -> Blockout_d_theta_SG_D_3_e0920/1

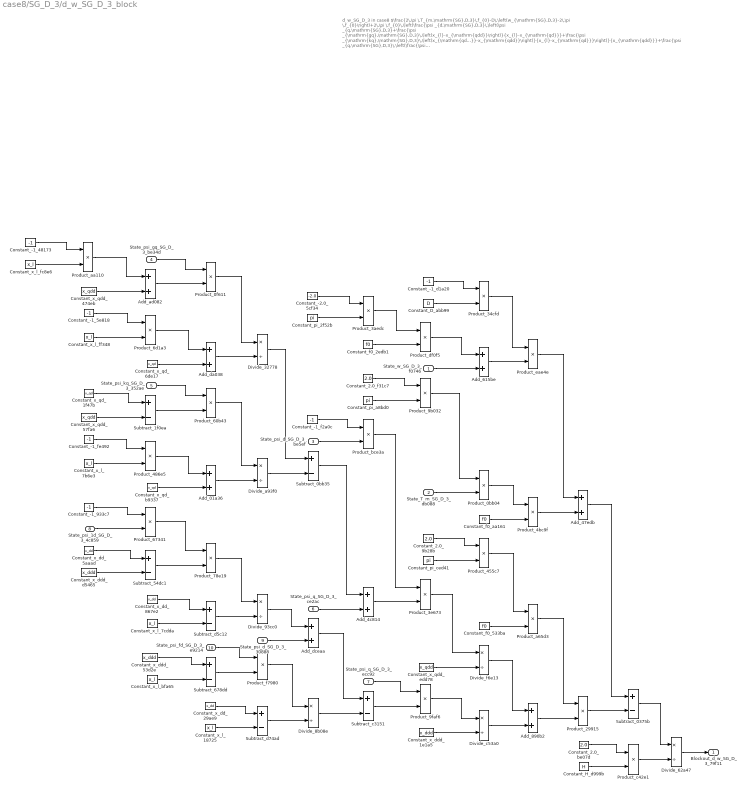
== system case8/SG_D_3/d_w_SG_D_3_block ==
  note: d_w_SG_D_3 in case8
      | $\frac{2\,\pi \,T_{m,\mathrm{SG},D,3}\,f_{0}-D\,\left(w_{\mathrm{SG},D,3}-2\,\pi \,f_{0}\right)+2\,\pi \,f_{0}\,\left(\frac{\psi _{d,\mathrm{SG},D,3}\,\left(\psi _{q,\mathrm{SG},D,3}+\frac{\psi _{\mathrm{gq},\mathrm{SG},D,3}\,\left(x_{l}-x_{\mathrm{qdd}}\right)}{x_{l}-x_{\mathrm{qd}}}+\frac{\psi _{\mathrm{kq},\mathrm{SG},D,3}\,\left(x_{\mathrm{qd}}-x_{\mathrm{qdd}}\right)}{x_{l}-x_{\mathrm{qd}}}\right)}{x_{\mathrm{qdd}}}+\frac{\psi _{q,\mathrm{SG},D,3}\,\left(\frac{\psi _{\mathrm{1d},\mathrm{SG},D,3}\,\left(x_{\mathrm{dd}}-x_{\mathrm{ddd}}\right)}{x_{\mathrm{dd}}-x_{l}}-\psi _{d,\mathrm{SG},D,3}+\frac{\psi _{\mathrm{fd},\mathrm{SG},D,3}\,\left(x_{\mathrm{ddd}}-x_{l}\right)}{x_{\mathrm{dd}}-x_{l}}\right)}{x_{\mathrm{ddd}}}\right)}{2\,H}$
      | Automatically generated on 2025-10-31 19:30:12 .
  State_w_SG_D_3_f0746 : Inport
  State_T_m_SG_D_3_db088 : Inport  Port=2
  State_psi_d_SG_D_3_be5ef : Inport  Port=3
  State_psi_gq_SG_D_3_be34d : Inport  Port=4
  State_psi_kq_SG_D_3_352ae : Inport  Port=5
  State_psi_q_SG_D_3_ce2ac : Inport  Port=6
  State_psi_q_SG_D_3_ecc92 : Inport  Port=7
  State_psi_1d_SG_D_3_4c859 : Inport  Port=8
  State_psi_d_SG_D_3_30888 : Inport  Port=9
  State_psi_fd_SG_D_3_e9214 : Inport  Port=10
  Add_01a36 : Sum
  Add_47edb : Sum
  Add_4c814 : Sum
  Add_615be : Sum
  Add_890b2 : Sum
  Add_ad082 : Sum
  Add_da038 : Sum
  Add_dceaa : Sum
  Constant_-1_48173 : Constant  Value=-1
  Constant_-1_5e818 : Constant  Value=-1
  Constant_-1_933c7 : Constant  Value=-1
  Constant_-1_d1a20 : Constant  Value=-1
  Constant_-1_f2a0c : Constant  Value=-1
  Constant_-1_fe492 : Constant  Value=-1
  Constant_-2.0_5cf34 : Constant  Value=-2.0
  Constant_2.0_9b28b : Constant  Value=2.0
  Constant_2.0_be07d : Constant  Value=2.0
  Constant_2.0_f31c7 : Constant  Value=2.0
  Constant_D_abb99 : Constant  Value=D
  Constant_H_d999b : Constant  Value=H
  Constant_f0_2edb1 : Constant  Value=f0
  Constant_f0_533ba : Constant  Value=f0
  Constant_f0_aa161 : Constant  Value=f0
  Constant_pi_2f52b : Constant  Value=pi
  Constant_pi_a8bd0 : Constant  Value=pi
  Constant_pi_ced41 : Constant  Value=pi
  Constant_x_dd_29ae9 : Constant  Value=x_dd
  Constant_x_dd_5aaad : Constant  Value=x_dd
  Constant_x_dd_867e2 : Constant  Value=x_dd
  Constant_x_ddd_1e1a5 : Constant  Value=x_ddd
  Constant_x_ddd_53d2e : Constant  Value=x_ddd
  Constant_x_ddd_d5465 : Constant  Value=x_ddd
  Constant_x_l_18725 : Constant  Value=x_l
  Constant_x_l_7b6e3 : Constant  Value=x_l
  Constant_x_l_7cdda : Constant  Value=x_l
  Constant_x_l_bfa65 : Constant  Value=x_l
  Constant_x_l_fc8e6 : Constant  Value=x_l
  Constant_x_l_ff348 : Constant  Value=x_l
  Constant_x_qd_1f47b : Constant  Value=x_qd
  Constant_x_qd_6de17 : Constant  Value=x_qd
  Constant_x_qd_b9337 : Constant  Value=x_qd
  Constant_x_qdd_474eb : Constant  Value=x_qdd
  Constant_x_qdd_57fa6 : Constant  Value=x_qdd
  Constant_x_qdd_edd78 : Constant  Value=x_qdd
  Divide_32778 : Product  Inputs=*/
  Divide_62a47 : Product  Inputs=*/
  Divide_8b08e : Product  Inputs=*/
  Divide_93cc0 : Product  Inputs=*/
  Divide_a93f0 : Product  Inputs=*/
  Divide_c53a0 : Product  Inputs=*/
  Divide_f6e13 : Product  Inputs=*/
  Product_0bb04 : Product
  Product_0f611 : Product
  Product_29915 : Product
  Product_34cfd : Product
  Product_3aedc : Product
  Product_3e673 : Product
  Product_455c7 : Product
  Product_486e5 : Product
  Product_4bc9f : Product
  Product_60b43 : Product
  Product_67341 : Product
  Product_6d1a3 : Product
  Product_78e19 : Product
  Product_9b032 : Product
  Product_9faf6 : Product
  Product_a65d3 : Product
  Product_aa110 : Product
  Product_bce3a : Product
  Product_c42e1 : Product
  Product_df0f5 : Product
  Product_eae4e : Product
  Product_f7980 : Product
  Subtract_0375b : Sum  Inputs=+-
  Subtract_0bb35 : Sum  Inputs=+-
  Subtract_1f0ea : Sum  Inputs=+-
  Subtract_54dc1 : Sum  Inputs=+-
  Subtract_678dd : Sum  Inputs=+-
  Subtract_c3151 : Sum  Inputs=+-
  Subtract_d5c12 : Sum  Inputs=+-
  Subtract_d74ad : Sum  Inputs=+-
  Blockout_d_w_SG_D_3_79f11 : Outport
  wires:
  Constant_x_qd_1f47b/1 -> Subtract_1f0ea/1
  Subtract_54dc1/1 -> Product_78e19/2
  Subtract_0375b/1 -> Divide_62a47/1
  Constant_-1_48173/1 -> Product_aa110/1
  Add_ad082/1 -> Product_0f611/2
  Constant_x_qdd_57fa6/1 -> Subtract_1f0ea/2
  Subtract_678dd/1 -> Product_f7980/2
  Constant_x_l_fc8e6/1 -> Product_aa110/2
  State_psi_d_SG_D_3_30888/1 -> Add_dceaa/2
  Add_da038/1 -> Divide_32778/2
  Constant_x_dd_867e2/1 -> Subtract_d5c12/1
  Constant_x_l_ff348/1 -> Product_6d1a3/2
  Constant_-1_d1a20/1 -> Product_34cfd/1
  Divide_8b08e/1 -> Subtract_c3151/2
  Constant_x_ddd_d5465/1 -> Subtract_54dc1/2
  Constant_x_qdd_474eb/1 -> Add_ad082/2
  Constant_pi_a8bd0/1 -> Product_9b032/2
  Product_aa110/1 -> Add_ad082/1
  Constant_-2.0_5cf34/1 -> Product_3aedc/1
  Constant_-1_5e818/1 -> Product_6d1a3/1
  Constant_2.0_9b28b/1 -> Product_455c7/1
  Product_3aedc/1 -> Product_df0f5/1
  Constant_-1_fe492/1 -> Product_486e5/1
  Subtract_0bb35/1 -> Add_4c814/1
  Constant_x_l_7b6e3/1 -> Product_486e5/2
  Constant_x_l_bfa65/1 -> Subtract_678dd/2
  Constant_-1_933c7/1 -> Product_67341/1
  State_psi_1d_SG_D_3_4c859/1 -> Product_67341/2
  Constant_x_dd_5aaad/1 -> Subtract_54dc1/1
  Product_67341/1 -> Product_78e19/1
  State_psi_gq_SG_D_3_be34d/1 -> Product_0f611/1
  Constant_x_qd_6de17/1 -> Add_da038/2
  Product_6d1a3/1 -> Add_da038/1
  State_psi_kq_SG_D_3_352ae/1 -> Product_60b43/1
  Subtract_1f0ea/1 -> Product_60b43/2
  Product_455c7/1 -> Product_a65d3/1
  Product_df0f5/1 -> Add_615be/1
  Product_486e5/1 -> Add_01a36/1
  State_psi_q_SG_D_3_ecc92/1 -> Product_9faf6/1
  Constant_x_qd_b9337/1 -> Add_01a36/2
  Constant_x_l_7cdda/1 -> Subtract_d5c12/2
  Constant_x_ddd_53d2e/1 -> Subtract_678dd/1
  Constant_x_l_18725/1 -> Subtract_d74ad/2
  Product_0f611/1 -> Divide_32778/1
  Product_60b43/1 -> Divide_a93f0/1
  Add_01a36/1 -> Divide_a93f0/2
  Product_78e19/1 -> Divide_93cc0/1
  Subtract_d5c12/1 -> Divide_93cc0/2
  Constant_2.0_f31c7/1 -> Product_9b032/1
  State_psi_fd_SG_D_3_e9214/1 -> Product_f7980/1
  Constant_x_dd_29ae9/1 -> Subtract_d74ad/1
  Divide_32778/1 -> Subtract_0bb35/1
  Product_f7980/1 -> Divide_8b08e/1
  Divide_a93f0/1 -> Subtract_0bb35/2
  Divide_93cc0/1 -> Add_dceaa/1
  Product_29915/1 -> Subtract_0375b/2
  Subtract_d74ad/1 -> Divide_8b08e/2
  Constant_pi_2f52b/1 -> Product_3aedc/2
  Constant_pi_ced41/1 -> Product_455c7/2
  Constant_-1_f2a0c/1 -> Product_bce3a/1
  State_psi_d_SG_D_3_be5ef/1 -> Product_bce3a/2
  State_psi_q_SG_D_3_ce2ac/1 -> Add_4c814/2
  Add_dceaa/1 -> Subtract_c3151/1
  Constant_f0_2edb1/1 -> Product_df0f5/2
  Product_bce3a/1 -> Product_3e673/1
  Add_4c814/1 -> Product_3e673/2
  Subtract_c3151/1 -> Product_9faf6/2
  Constant_D_abb99/1 -> Product_34cfd/2
  State_w_SG_D_3_f0746/1 -> Add_615be/2
  Product_9b032/1 -> Product_0bb04/1
  State_T_m_SG_D_3_db088/1 -> Product_0bb04/2
  Product_3e673/1 -> Divide_f6e13/1
  Constant_x_qdd_edd78/1 -> Divide_f6e13/2
  Product_9faf6/1 -> Divide_c53a0/1
  Constant_x_ddd_1e1a5/1 -> Divide_c53a0/2
  Product_34cfd/1 -> Product_eae4e/1
  Add_615be/1 -> Product_eae4e/2
  Product_0bb04/1 -> Product_4bc9f/1
  Constant_f0_aa161/1 -> Product_4bc9f/2
  Constant_f0_533ba/1 -> Product_a65d3/2
  Divide_f6e13/1 -> Add_890b2/1
  Divide_c53a0/1 -> Add_890b2/2
  Product_eae4e/1 -> Add_47edb/1
  Product_4bc9f/1 -> Add_47edb/2
  Product_a65d3/1 -> Product_29915/1
  Add_890b2/1 -> Product_29915/2
  Add_47edb/1 -> Subtract_0375b/1
  Constant_2.0_be07d/1 -> Product_c42e1/1
  Constant_H_d999b/1 -> Product_c42e1/2
  Product_c42e1/1 -> Divide_62a47/2
  Divide_62a47/1 -> Blockout_d_w_SG_D_3_79f11/1

== system case8/SG_D_3/i_d_SG_D_3_block ==
  note: i_d_SG_D_3 in case8
      | $\frac{\sin\left(\theta _{\mathrm{SG},D,3}\right)\,\left(\frac{\psi _{\mathrm{1d},\mathrm{SG},D,3}\,\left(x_{\mathrm{dd}}-x_{\mathrm{ddd}}\right)}{x_{\mathrm{dd}}-x_{l}}-\psi _{d,\mathrm{SG},D,3}+\frac{\psi _{\mathrm{fd},\mathrm{SG},D,3}\,\left(x_{\mathrm{ddd}}-x_{l}\right)}{x_{\mathrm{dd}}-x_{l}}\right)}{x_{\mathrm{ddd}}}-\frac{\cos\left(\theta _{\mathrm{SG},D,3}\right)\,\left(\psi _{q,\mathrm{SG},D,3}+\frac{\psi _{\mathrm{gq},\mathrm{SG},D,3}\,\left(x_{l}-x_{\mathrm{qdd}}\right)}{x_{l}-x_{\mathrm{qd}}}+\frac{\psi _{\mathrm{kq},\mathrm{SG},D,3}\,\left(x_{\mathrm{qd}}-x_{\mathrm{qdd}}\right)}{x_{l}-x_{\mathrm{qd}}}\right)}{x_{\mathrm{qdd}}}$
      | Automatically generated on 2025-10-31 19:30:18 .
  State_psi_gq_SG_D_3_8b9f6 : Inport
  State_psi_kq_SG_D_3_4b8d1 : Inport  Port=2
  State_psi_q_SG_D_3_5ee11 : Inport  Port=3
  State_theta_SG_D_3_341cf : Inport  Port=4
  State_psi_1d_SG_D_3_83346 : Inport  Port=5
  State_psi_d_SG_D_3_2ac54 : Inport  Port=6
  State_psi_fd_SG_D_3_bd64a : Inport  Port=7
  State_theta_SG_D_3_d9be7 : Inport  Port=8
  Add_7cf07 : Sum
  Add_84aaf : Sum
  Add_bbed2 : Sum
  Add_c4075 : Sum
  Add_d7b90 : Sum
  Constant_-1_20889 : Constant  Value=-1
  Constant_-1_430a1 : Constant  Value=-1
  Constant_-1_59f18 : Constant  Value=-1
  Constant_-1_61ea2 : Constant  Value=-1
  Constant_-1_d91f5 : Constant  Value=-1
  Constant_x_dd_02b66 : Constant  Value=x_dd
  Constant_x_dd_7521d : Constant  Value=x_dd
  Constant_x_dd_ccafd : Constant  Value=x_dd
  Constant_x_ddd_33dcb : Constant  Value=x_ddd
  Constant_x_ddd_653f3 : Constant  Value=x_ddd
  Constant_x_ddd_f7407 : Constant  Value=x_ddd
  Constant_x_l_1de9d : Constant  Value=x_l
  Constant_x_l_2292f : Constant  Value=x_l
  Constant_x_l_3871c : Constant  Value=x_l
  Constant_x_l_91d21 : Constant  Value=x_l
  Constant_x_l_db051 : Constant  Value=x_l
  Constant_x_l_f71a3 : Constant  Value=x_l
  Constant_x_qd_103bf : Constant  Value=x_qd
  Constant_x_qd_6dd61 : Constant  Value=x_qd
  Constant_x_qd_84278 : Constant  Value=x_qd
  Constant_x_qdd_89d44 : Constant  Value=x_qdd
  Constant_x_qdd_a6af7 : Constant  Value=x_qdd
  Constant_x_qdd_ab01a : Constant  Value=x_qdd
  Divide_170c6 : Product  Inputs=*/
  Divide_37ff2 : Product  Inputs=*/
  Divide_539e1 : Product  Inputs=*/
  Divide_c2177 : Product  Inputs=*/
  Divide_cbb18 : Product  Inputs=*/
  Divide_d8c32 : Product  Inputs=*/
  MathFunc_cos_7e8fe : Trigonometry  Operator=cos
  MathFunc_sin_58e74 : Trigonometry
  Product_08b4c : Product
  Product_123ee : Product
  Product_15e6b : Product
  Product_244c5 : Product
  Product_24ea4 : Product
  Product_850b7 : Product
  Product_8e41a : Product
  Product_b3f82 : Product
  Product_bb1c8 : Product
  Product_c4a4d : Product
  Product_f18a0 : Product
  Subtract_36a3d : Sum  Inputs=+-
  Subtract_405bc : Sum  Inputs=+-
  Subtract_54415 : Sum  Inputs=+-
  Subtract_639a1 : Sum  Inputs=+-
  Subtract_768bf : Sum  Inputs=+-
  Subtract_81571 : Sum  Inputs=+-
  Subtract_86b27 : Sum  Inputs=+-
  Subtract_af1d2 : Sum  Inputs=+-
  Blockout_i_d_SG_D_3_d7069 : Outport
  wires:
  Constant_x_qd_103bf/1 -> Subtract_768bf/1
  Subtract_86b27/1 -> Blockout_i_d_SG_D_3_d7069/1
  Constant_-1_61ea2/1 -> Product_8e41a/1
  Constant_x_l_f71a3/1 -> Product_08b4c/2
  Constant_x_qdd_ab01a/1 -> Add_c4075/2
  Constant_x_qdd_a6af7/1 -> Subtract_768bf/2
  Constant_x_l_3871c/1 -> Product_8e41a/2
  Divide_539e1/1 -> Subtract_86b27/1
  Product_8e41a/1 -> Add_c4075/1
  Constant_x_ddd_f7407/1 -> Subtract_54415/2
  Constant_-1_20889/1 -> Product_08b4c/1
  Constant_-1_d91f5/1 -> Product_123ee/1
  Constant_x_l_91d21/1 -> Product_123ee/2
  State_psi_1d_SG_D_3_83346/1 -> Product_24ea4/2
  State_psi_gq_SG_D_3_8b9f6/1 -> Product_850b7/1
  Product_24ea4/1 -> Product_b3f82/1
  Add_c4075/1 -> Product_850b7/2
  Product_08b4c/1 -> Add_d7b90/1
  Constant_x_qd_84278/1 -> Add_d7b90/2
  State_psi_kq_SG_D_3_4b8d1/1 -> Product_15e6b/1
  Subtract_36a3d/1 -> Divide_cbb18/2
  Subtract_768bf/1 -> Product_15e6b/2
  Product_123ee/1 -> Add_7cf07/1
  Constant_x_ddd_653f3/1 -> Subtract_639a1/1
  Constant_x_qd_6dd61/1 -> Add_7cf07/2
  Constant_-1_59f18/1 -> Product_24ea4/1
  Constant_x_dd_02b66/1 -> Subtract_54415/1
  Product_850b7/1 -> Divide_d8c32/1
  Add_d7b90/1 -> Divide_d8c32/2
  Product_15e6b/1 -> Divide_170c6/1
  Add_7cf07/1 -> Divide_170c6/2
  Divide_cbb18/1 -> Subtract_81571/2
  Subtract_54415/1 -> Product_b3f82/2
  State_theta_SG_D_3_341cf/1 -> MathFunc_cos_7e8fe/1
  Constant_x_dd_ccafd/1 -> Subtract_405bc/1
  Product_bb1c8/1 -> Product_c4a4d/1
  Constant_x_l_1de9d/1 -> Subtract_405bc/2
  Add_84aaf/1 -> Subtract_81571/1
  Constant_x_l_db051/1 -> Subtract_639a1/2
  State_theta_SG_D_3_d9be7/1 -> MathFunc_sin_58e74/1
  Divide_d8c32/1 -> Subtract_af1d2/1
  Add_bbed2/1 -> Product_bb1c8/2
  Divide_170c6/1 -> Subtract_af1d2/2
  Product_b3f82/1 -> Divide_37ff2/1
  Subtract_405bc/1 -> Divide_37ff2/2
  State_psi_fd_SG_D_3_bd64a/1 -> Product_244c5/1
  Divide_c2177/1 -> Subtract_86b27/2
  Subtract_639a1/1 -> Product_244c5/2
  Constant_x_dd_7521d/1 -> Subtract_36a3d/1
  Subtract_af1d2/1 -> Add_bbed2/1
  Constant_x_l_2292f/1 -> Subtract_36a3d/2
  Constant_-1_430a1/1 -> Product_bb1c8/1
  State_psi_q_SG_D_3_5ee11/1 -> Add_bbed2/2
  Divide_37ff2/1 -> Add_84aaf/1
  State_psi_d_SG_D_3_2ac54/1 -> Add_84aaf/2
  Product_244c5/1 -> Divide_cbb18/1
  MathFunc_cos_7e8fe/1 -> Product_c4a4d/2
  MathFunc_sin_58e74/1 -> Product_f18a0/2
  Subtract_81571/1 -> Product_f18a0/1
  Product_c4a4d/1 -> Divide_539e1/1
  Constant_x_qdd_89d44/1 -> Divide_539e1/2
  Product_f18a0/1 -> Divide_c2177/1
  Constant_x_ddd_33dcb/1 -> Divide_c2177/2
